simulink model "ModeloSimulacion"  (R2023a)
settings: Solver=VariableStepAuto  StartTime=0.0  StopTime=10.0  RelTol=1e-3
undefined symbols (not defined in the file): sampleTime, scanAngles
libraries: mobileRoboticsLib x4, simulink x2, robotalgslib x2
settings Model: Creator=John_117  LastModifiedBy=John_117

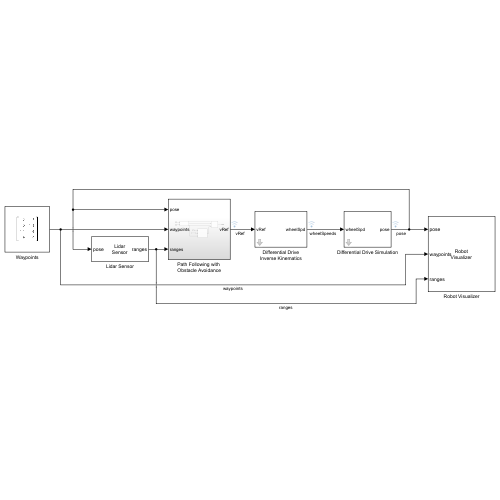
[thumbnail: Simulink's stored preview of the top-level diagram]
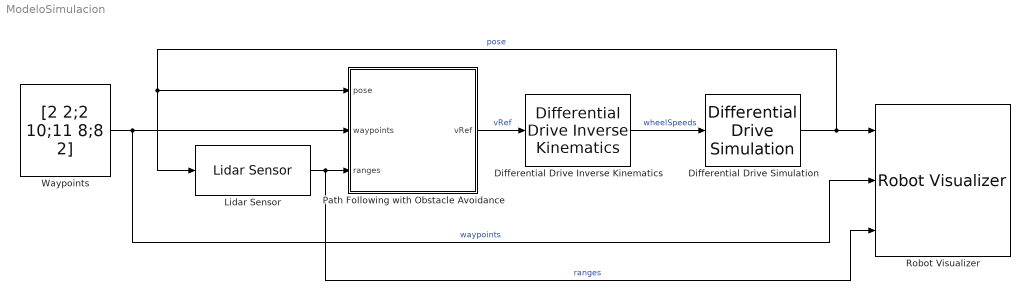
== system ModeloSimulacion ==
  Differential Drive Inverse Kinematics : mobileRoboticsLib/Kinematic Models/Differential Drive/Differential Drive Inverse Kinematics  wheelRadius=R  wheelBase=L
      settings: SourceProductName=Mobile Robotics Simulation Toolbox
  Differential Drive Simulation : mobileRoboticsLib/Kinematic Models/Differential Drive/Differential Drive Simulation  wheelRadius=R  wheelBase=L  initX=2  initY=2  initAngle=0  Ts=sampleTime
      settings: SourceProductName=Mobile Robotics Simulation Toolbox
  Lidar Sensor : mobileRoboticsLib/Environments/Lidar Sensor  mapName=map  sensorOffset=scanSensorOffset  scanAngles=scanAngles  maxRange=scanMaxRange
      settings: SourceProductName=Mobile Robotics Simulation Toolbox
  Path Following with Obstacle Avoidance : Subsystem
  Robot Visualizer : mobileRoboticsLib/Environments/Robot Visualizer  Priority=99  robotRadius=0  mapName=map  showTrajectory=on  hasWaypoints=on  hasLidar=on  sensorOffset=scanSensorOffset  scanAngles=scanAngles  hasObjDetector=off  objDetectorOffset=[ 0, 0 ]  objDetectorAngle=0  objDetectorFOV=0  objDetectorMaxRange=0  objectColors=0  objectMarkers='s'
  Waypoints : Constant  Value=[2 2;2 10;11 8;8 2]
  wires:
  Waypoints/1 -> Path Following with Obstacle Avoidance/2(waypoints), Robot Visualizer/2  "waypoints"
  Path Following with Obstacle Avoidance/1(vRef) -> Differential Drive Inverse Kinematics/1  "vRef"
  Lidar Sensor/1 -> Robot Visualizer/3, Path Following with Obstacle Avoidance/3(ranges)  "ranges"
  Differential Drive Simulation/1 -> Robot Visualizer/1, Path Following with Obstacle Avoidance/1(pose), Lidar Sensor/1  "pose"
  Differential Drive Inverse Kinematics/1 -> Differential Drive Simulation/1  "wheelSpeeds"

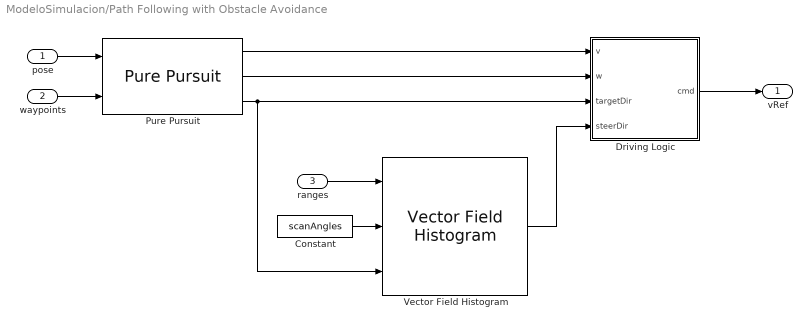
== system ModeloSimulacion/Path Following with Obstacle Avoidance ==
  pose : Inport
  waypoints : Inport  Port=2
  ranges : Inport  Port=3
  Constant : Constant  Value=scanAngles
  Driving Logic : Subsystem
  Pure Pursuit : robotalgslib/Pure Pursuit  DesiredLinearVelocity=0.75  MaxAngularVelocity=1.5  LookaheadDistance=0.5  TargetDirPort=on  SimulateUsing=Interpreted execution
  Vector Field Histogram : robotalgslib/Vector Field Histogram  NumAngularSectors=36  DistanceLimits=[ 0.05, 3 ]  HistogramThresholds=[ 5, 10 ]  RobotRadius=L  SafetyDistance=L  MinTurningRadius=0.25  SimulateUsing=Interpreted execution  TargetDirectionWeight=5  CurrentDirectionWeight=2  PreviousDirectionWeight=2
  vRef : Outport  VectorParamsAs1DForOutWhenUnconnected=off
  wires:
  pose/1 -> Pure Pursuit/1
  Pure Pursuit/3 -> Driving Logic/3(targetDir), Vector Field Histogram/3
  Pure Pursuit/1 -> Driving Logic/1(v)
  Constant/1 -> Vector Field Histogram/2
  Vector Field Histogram/1 -> Driving Logic/4(steerDir)
  ranges/1 -> Vector Field Histogram/1
  waypoints/1 -> Pure Pursuit/2
  Pure Pursuit/2 -> Driving Logic/2(w)
  Driving Logic/1(cmd) -> vRef/1

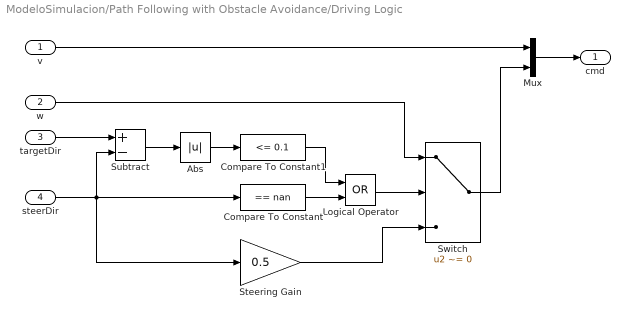
== system ModeloSimulacion/Path Following with Obstacle Avoidance/Driving Logic ==
  v : Inport
  w : Inport  Port=2
  targetDir : Inport  Port=3
  steerDir : Inport  Port=4
  Abs : Abs  SaturateOnIntegerOverflow=off
  Compare To Constant : simulink/Logic and Bit Operations/Compare To Constant  relop===  const=nan  OutDataTypeStr=boolean
  Compare To Constant1 : simulink/Logic and Bit Operations/Compare To Constant  relop=<=  const=0.1  OutDataTypeStr=boolean
  Logical Operator : Logic  Operator=OR  AllPortsSameDT=off  OutDataTypeStr=boolean
  Mux : Mux  Inputs=2
  Steering Gain : Gain  Gain=0.5
  Subtract : Sum  Inputs=+-
  Switch : Switch  Criteria=u2 ~= 0  SaturateOnIntegerOverflow=off  InputSameDT=off
  cmd : Outport  VectorParamsAs1DForOutWhenUnconnected=off
  wires:
  v/1 -> Mux/1
  steerDir/1 -> Steering Gain/1, Subtract/2, Compare To Constant/1
  Compare To Constant/1 -> Logical Operator/2
  targetDir/1 -> Subtract/1
  Subtract/1 -> Abs/1
  Abs/1 -> Compare To Constant1/1
  Compare To Constant1/1 -> Logical Operator/1
  Mux/1 -> cmd/1
  Logical Operator/1 -> Switch/2
  w/1 -> Switch/1
  Switch/1 -> Mux/2
  Steering Gain/1 -> Switch/3
